simulink model "Linear_pole_place"  (R2015b)
settings: Solver=VariableStepAuto  StartTime=0.0  StopTime=300  RelTol=1e-3
undefined symbols (not defined in the file): A, B, l
settings Model: Creator=Pramod  LastModifiedBy=Pramod

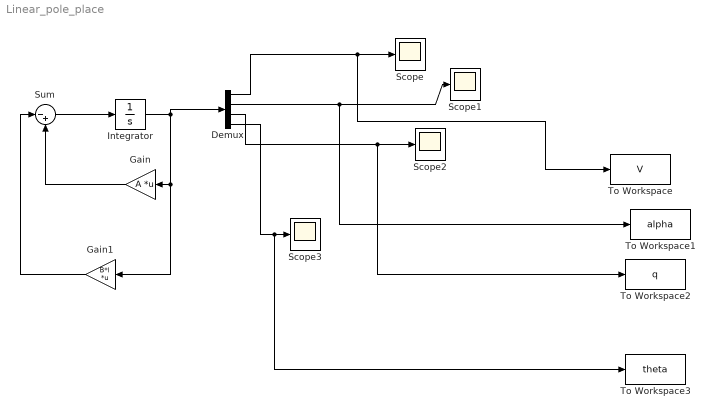
== system Linear_pole_place ==
  Demux : Demux
  Gain : Gain  Gain=A  Multiplication=Matrix(K*u)
  Gain1 : Gain  Gain=B*l  Multiplication=Matrix(K*u)
  Integrator : Integrator  InitialCondition="[39.5514    0.0872   -0.0000    1.3099]"
  Scope{,1..3} (4 alike) : Scope
  Sum : Sum  Inputs=|-+
  To Workspace : ToWorkspace  VariableName=V  SaveFormat=Timeseries  SampleTime=-1
  To Workspace1 : ToWorkspace  VariableName=alpha  SaveFormat=Timeseries  SampleTime=-1
  To Workspace2 : ToWorkspace  VariableName=q  SaveFormat=Timeseries  SampleTime=-1
  To Workspace3 : ToWorkspace  VariableName=theta  SaveFormat=Timeseries  SampleTime=-1
  wires:
  Integrator/1 -> Gain1/1, Gain/1, Demux/1
  Gain/1 -> Sum/2
  Sum/1 -> Integrator/1
  Demux/1 -> To Workspace/1, Scope/1
  Demux/2 -> To Workspace1/1, Scope1/1
  Demux/3 -> To Workspace2/1, Scope2/1
  Demux/4 -> To Workspace3/1, Scope3/1
  Gain1/1 -> Sum/1
